simulink model "SimHydraulics_Actuation_System_BH"  (R2013a)
settings: Solver=ode15s  StartTime=0.0  StopTime=10.0  RelTol=1e-3
model workspace (MAT data in the model file):
  cylinderGray = [0.6 0.6 0.6]
  darkOrange = [0.8 0.5 0]
  glassBlue = [0.2 0.2 1]
  gray = [0.3 0.3 0.3]
  orange = [0.8 0.65 0]
  pistonGray = [0.4 0.4 0.4]
  tireBlack = [0.1 0.1 0.1]
  wheelGray = [0.6 0.6 0.6]
  yellow = [0.8 0.8 0]
  rhoGlass = 2500
  rhoRubber = 1500
  rhoSteel = 7800
libraries: sh_lib x5, fl_lib x4, nesl_utility x3, Tilt_Actuator_Lib x1
Description:
  | Copyright 2013 The MathWorks, Inc.
settings Model: Creator=smiller  LastModifiedBy=smiller
settings OptimizationCC: ExpressionDepthLimit=2147483647
settings ExplorerConfigSet: InternalSimMechanicsExplorerSettings="<ExplorerConfiguration><canonicalview>default</canonicalview><TilePanel><TileInfo><Tiles Columns=\"1\" Count=\"1\" Rows=\"1\"><Column Left=\"2\" Weight=\"1\"/><Column Left=\"603\"/><Row Top=\"2\" Weight=\"1\"/><Row Top=\"639\"/><Tile Height=\"1\" Width=\"1\" X=\"0\" Y=\"0\"/></Tiles></TileInfo><SceneInfo><SceneViewer><BGColor><R>0.60000002384185791</R><G>0.60000002384185791</G><B>0.60000002384185791</B></BGColor><Camera><Position><X>4.2115543563123818</X><Y>-3.1200241025244861</Y><Z>-9.457800303521676</Z></Position><Center><X>1.7410059792522423</X><Y>1.9057541085977436</Y><Z>0.10201332843757704</Z></Center><Up><X>-0.12825683907994126</X><Y>-0.89109326109265186</Y><Z>0.4353194037307378</Z></Up><Left>-2.6694327592849731</Left><Right>2.6694327592849731</Right><Bottom>-4.914561080932617</Bottom><Top>4.914561080932617</Top></Camera></SceneViewer></SceneInfo></TilePanel></ExplorerConfiguration>"

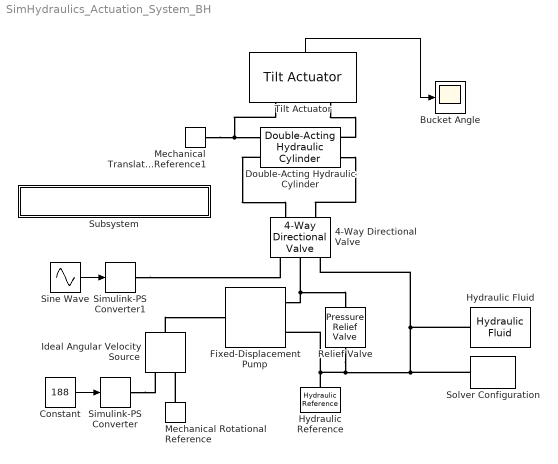
== system SimHydraulics_Actuation_System_BH ==
  4-Way Directional Valve : sh_lib/Valves/Directional Valves/4-Way Directional Valve  mdl_type=1  area_max=5e-04 m^2  opening_max=0.005 m  opening_tab="[  -0.002 0 0.005 0.015 ] m"  area_tab="[  1e-12 4e-12 1e-05 1.02e-05 ] m^2"  pressure_tab="[  -5e+06 -2e+06 2e+06 5e+06 ] Pa"  flow_rate_tab="[  -1e-12 -6e-14 6e+12 1e+11 ; -8e-08 -4e-08 4e+06 8e+06 ; -0.0025 -0.00103 0.001 0.0024 ; -0.00258 -0.001032 0.00106 0.00247 ; ] m^3/s"  interp_method=1  extrap_method=1  C_d=0.7  x_0_P_A=0 m  x_0_P_B=0 m  x_0_A_T=0 m  x_0_B_T=0 m  Re_cr=12  A_leak=1e-12 m^2  LocalVarLogging=[]
  Bucket Angle : Scope
      settings: TimeRange=10  YMin=-80  YMax=0
  Constant : Constant  Value=188
  Double-Acting Hydraulic Cylinder : sh_lib/Hydraulic Cylinders/Double-Acting Hydraulic Cylinder  area_A=0.125 m^2  area_B=0.125 m^2  stroke=0.5 m  init_pos=0 m  dead_vol_A=1e-04 m^3  dead_vol_B=1e-04 m^3  init_pressure_A=0 Pa  init_pressure_B=0 Pa  k_sh=1.4  stiff=1e9 N/m  D=150 N/(m/s)  or=1  LocalVarLogging=[]
  Fixed-Displacement Pump : sh_lib/Pumps and Motors/Fixed-Displacement Pump  D=5e-04 m^3/rad  efficiency_vol=0.92  efficiency_tot=0.8  pr_nominal=1e+7 Pa  w_nominal=188 rad/s  visc_nominal=18 cSt  pump_delivery_Log=off  leakage_flow_Log=off  torque_Log=off  power_hyd_Log=off  pressure_diff_Log=off  shaft_ang_vel_Log=off  LocalVarNames=|pump_delivery|leakage_flow|torque|power_hyd|pressure_diff|shaft_ang_vel  LocalVarDescs=|Pump delivery (m^3/s)|Leakage flow rate (m^3/s)|Driving shaft torque (N*m)|Output flow power (W)|Pressure differential (Pa)|Driving shaft angular velocity (rad/s)  LocalVarLogging=[0 0 0 0 0 0]
  Hydraulic Reference : fl_lib/Hydraulic/Hydraulic Elements/Hydraulic Reference  q_Log=off  LocalVarNames=|q  LocalVarDescs=|q  LocalVarLogging=[]
  Hydraulic Fluid : sh_lib/Hydraulic Utilities/Hydraulic Fluid  DataSource=1  SelFluid=1  SysTemp=60 c  TrapAir=0.005  ViscDerFactor=1  LocalVarLogging=[]
  Ideal Angular Velocity Source : fl_lib/Mechanical/Mechanical Sources/Ideal Angular Velocity Source  w_Log=off  t_Log=off  LocalVarNames=|torque|rel_velocity|power  LocalVarDescs=|Torque (N*m)|Relative velocity (rad/s)|Power generated by the sourcec(W)  LocalVarLogging=[0 0 0]
  Mechanical Rotational Reference : fl_lib/Mechanical/Rotational Elements/Mechanical Rotational Reference  t_Log=off  LocalVarNames=|t  LocalVarDescs=|t  LocalVarLogging=[]
  Mechanical Translational Reference1 : fl_lib/Mechanical/Translational Elements/Mechanical Translational Reference  Tag=Factory Generic  f_Log=off  LocalVarNames=|f  LocalVarDescs=|f  LocalVarLogging=[]
  Relief Valve : sh_lib/Valves/Pressure Control Valves/Pressure Relief Valve  area_max=2e-4 m^2  pres_set=3e7 Pa  reg_range=3e6 Pa  C_d=0.7  Re_cr=12  A_leak=1e-12 m^2  flow_rate_Log=off  pr_drop_Log=off  power_Log=off  area_Log=off  Re_Log=off  LocalVarNames=|flow_rate|pr_drop|power|area|Re  LocalVarDescs=|Flow rate through the valve (m^3/s)|Pressure differential across the valve (Pa)|Hydraulic loss power (W)|Instantaneous passage area (m^2)|Reynolds number  LocalVarLogging=[0 0 0 0 0]
  Simulink-PS Converter : nesl_utility/Simulink-PS Converter  PhysicalDomain=network_engine_domain  SubClassName=ps_input  LeftPortType=input  RightPortType=output  PseudoPeriodic=off  Frequencies=[]  NoiseDistribution=none  NoiseParameters=[]  Unit=rad/s  AffineConversion=off  InputFiltering=off  SimscapeFilterOrder=1  InputFilterTimeConstant=.001  UdotUserProvided=0
  Simulink-PS Converter1 : nesl_utility/Simulink-PS Converter  PhysicalDomain=network_engine_domain  SubClassName=ps_input  LeftPortType=input  RightPortType=output  PseudoPeriodic=off  Frequencies=[]  NoiseDistribution=none  NoiseParameters=[]  Unit=m  AffineConversion=off  InputFiltering=off  SimscapeFilterOrder=1  InputFilterTimeConstant=.001  UdotUserProvided=0
  Sine Wave : Sin  Amplitude=3e-3  SampleTime=0
  Solver Configuration : nesl_utility/Solver Configuration  PhysicalDomain=network_engine_domain  SubClassName=solver  LeftPortType=input  RightPortType=generic  Accelerate=off  Tones=[]  Harmonics=[]  SimulateNoise=off  Profile=off  UseLocalSampling=off  EnableSwitchedLinearOptims=on  FrequencyDomain=off  UseCCode=off  UseNewInitialization=off  DoDC=off  ResidualTolerance=1e-9  UseLocalSolver=off  LocalSolverChoice=NE_BACKWARD_EULER_ADVANCER  LocalSolverSampleTime=.001  DoFixedCost=off  MaxNonlinIter=12  MaxModeIter=2  LinearAlgebra=Sparse  DelaysMemoryBudget=1024
  Subsystem : Subsystem
      settings: OpenFcn=simlog.Relief_Valve.A.p.plot;
      mask Display: text(0.02,0.5,'>> simlog.Relief_Valve.A.p.plot;');
  Tilt Actuator : Tilt_Actuator_Lib/Tilt Actuator  SystemSampleTime=-1
  wires:
  Constant/1 -> Simulink-PS Converter/1
  Sine Wave/1 -> Simulink-PS Converter1/1
  Tilt Actuator/1 -> Bucket Angle/1
  connections:
  Relief Valve/LConn1 -- Fixed-Displacement Pump/RConn1 -- 4-Way Directional Valve/RConn2
  Solver Configuration/RConn1 -- Hydraulic Reference/LConn1 -- Fixed-Displacement Pump/RConn2 -- Relief Valve/RConn1 -- 4-Way Directional Valve/RConn3 -- Hydraulic Fluid/RConn1
  Mechanical Translational Reference1/LConn1 -- Tilt Actuator/LConn1 -- Double-Acting Hydraulic Cylinder/LConn1
  Ideal Angular Velocity Source/LConn1 -- Fixed-Displacement Pump/LConn1
  Mechanical Rotational Reference/LConn1 -- Ideal Angular Velocity Source/RConn2
  Double-Acting Hydraulic Cylinder/LConn2 -- 4-Way Directional Valve/LConn1
  Double-Acting Hydraulic Cylinder/RConn2 -- 4-Way Directional Valve/LConn2
  Simulink-PS Converter1/RConn1 -- 4-Way Directional Valve/RConn1
  Simulink-PS Converter/RConn1 -- Ideal Angular Velocity Source/RConn1
  Tilt Actuator/LConn2 -- Double-Acting Hydraulic Cylinder/RConn1

== system SimHydraulics_Actuation_System_BH/Subsystem ==
